simulink model "Pendel_01"  (Simulink 10.1)
settings: Solver=ode45  StartTime=0.0  StopTime=10.0  RelTol=1e-3  EnableMultiTasking=on
values from neighbouring files (symbols this model uses):
  A1 = [0   -g/L ... (first row only)    [test_simulink.m]    (also in ueb_simulink_Pendel.m)
  B1 = [0 0]'    [test_simulink.m]    (also in ueb_simulink_Pendel.m)
  C1 = [1 0 ... (first row only)    [test_simulink.m]    (also in ueb_simulink_Pendel.m)
  D1 = [0 0]'    [test_simulink.m]    (also in ueb_simulink_Pendel.m)
  g = 9.81    [test_simulink.m]    (also in ueb_simulink_Pendel.m)
  L = 84e-6/2    (= 4.2e-05)    [bldc_motor.m]    (also in test_simulink.m = 10; ueb_simulink_Pendel.m = 10)
  Omega_0 = 0    [test_simulink.m]    (also in ueb_simulink_Pendel.m)
  Phi_0 = 60*pi/180    (= 1.0471975512)    [test_simulink.m]    (also in ueb_simulink_Pendel.m)
  x1_0 = [Omega_0 Phi_0]'    [test_simulink.m]    (also in ueb_simulink_Pendel.m)
settings Model: Creator=dep02378  LastModifiedBy=Horst
settings DataIOCC: LimitDataPoints=on  SignalLoggingSaveFormat=ModelDataLogs
settings OptimizationCC: ExpressionDepthLimit=2147483647
settings DebuggingCC: SolverPrmCheckMsg=warning  FcnCallInpInsideContextMsg=warning  StateNameClashWarn=warning
settings GRTTargetCC: CombineOutputUpdateFcns=on  GRTInterface=off

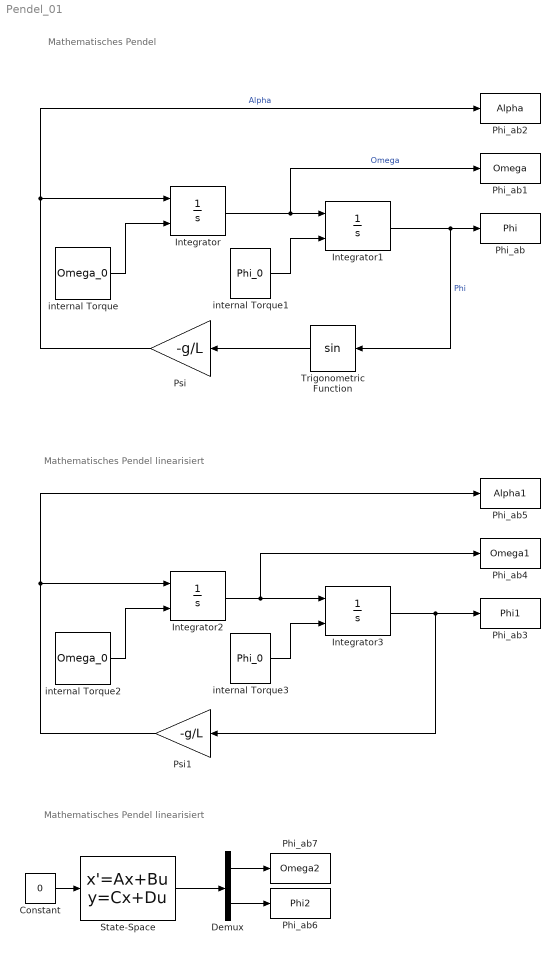
== system Pendel_01 ==
  note: Mathematisches Pendel
  note: Mathematisches Pendel linearisiert
  note: Mathematisches Pendel linearisiert
  Constant : Constant  Value=0
  Demux : Demux  Outputs=2
  Integrator{,1..3} (4 alike) : Integrator  InitialConditionSource=external
  Phi_ab : ToWorkspace  VariableName=Phi  SampleTime=-1
  Phi_ab1 : ToWorkspace  VariableName=Omega  SampleTime=-1
  Phi_ab2 : ToWorkspace  VariableName=Alpha  SampleTime=-1
  Phi_ab3 : ToWorkspace  VariableName=Phi1  SampleTime=-1
  Phi_ab4 : ToWorkspace  VariableName=Omega1  SampleTime=-1
  Phi_ab5 : ToWorkspace  VariableName=Alpha1  SampleTime=-1
  Phi_ab6 : ToWorkspace  VariableName=Phi2  SampleTime=-1
  Phi_ab7 : ToWorkspace  VariableName=Omega2  SampleTime=-1
  Psi : Gain  Gain=-g/L
  Psi1 : Gain  Gain=-g/L
  State-Space : StateSpace  A=A1  B=B1  C=C1  D=D1  InitialCondition=x1_0
  Trigonometric Function : Trigonometry
  internal Torque : Constant  Value=Omega_0
  internal Torque1 : Constant  Value=Phi_0
  internal Torque2 : Constant  Value=Omega_0
  internal Torque3 : Constant  Value=Phi_0
  wires:
  Integrator/1 -> Integrator1/1, Phi_ab1/1  "Omega"
  Integrator1/1 -> Phi_ab/1, Trigonometric Function/1  "Phi"
  Trigonometric Function/1 -> Psi/1
  internal Torque/1 -> Integrator/2
  internal Torque1/1 -> Integrator1/2
  Psi/1 -> Integrator/1, Phi_ab2/1  "Alpha"
  Integrator2/1 -> Integrator3/1, Phi_ab4/1
  Integrator3/1 -> Phi_ab3/1, Psi1/1
  internal Torque2/1 -> Integrator2/2
  internal Torque3/1 -> Integrator3/2
  Psi1/1 -> Integrator2/1, Phi_ab5/1
  Constant/1 -> State-Space/1
  State-Space/1 -> Demux/1
  Demux/2 -> Phi_ab6/1
  Demux/1 -> Phi_ab7/1
